simulink model "test_codegen_sim_02"  (Simulink 7.9)
settings: Solver=ode45  StartTime=0.0  StopTime=10.0  RelTol=1e-3
libraries: mpt_sim x1
settings Model: Creator=mato  LastModifiedBy=mato

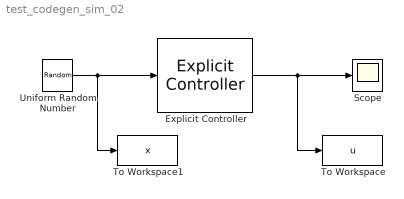
== system test_codegen_sim_02 ==
  Explicit Controller : mpt_sim/Explicit Controller
  Scope : Scope
      settings: TimeRange=10
  To Workspace : ToWorkspace  VariableName=u  SampleTime=-1
  To Workspace1 : ToWorkspace  VariableName=x  SampleTime=-1
  Uniform Random Number : UniformRandomNumber  Seed=[0;1]  SampleTime=1
  wires:
  Explicit Controller/1 -> Scope/1, To Workspace/1
  Uniform Random Number/1 -> Explicit Controller/1, To Workspace1/1
